simulink model "MidEval3"  (R2022b)
settings: Solver=VariableStepAuto  StartTime=0.0  StopTime=10.0  MaxStep=1e-3  RelTol=1e-4
model workspace (MAT data in the model file):
  DataStore = Simulink.Parameter
  DataStore.Value = [1 0 0 1 0 0 0 1 1 0 0 1 ... (2240 elements, 2240x1)]
  DataStore.DataType = 'auto'
  DataStore.Complexity = 'real'
  DataStore.Dimensions = [2240 1]
  Freq = Simulink.Parameter
  Freq.Value = 2000
  Freq.DataType = 'auto'
  Freq.Complexity = 'real'
  Freq.Dimensions = [1 1]
  Freq2 = Simulink.Parameter
  Freq2.Value = 6000000
  Freq2.DataType = 'auto'
  Freq2.Complexity = 'real'
  Freq2.Dimensions = [1 1]
  Freq3 = Simulink.Parameter
  Freq3.Value = 3000000
  Freq3.DataType = 'auto'
  Freq3.Complexity = 'real'
  Freq3.Dimensions = [1 1]
  Freq4 = Simulink.Parameter
  Freq4.Value = 10000000
  Freq4.DataType = 'auto'
  Freq4.Complexity = 'real'
  Freq4.Dimensions = [1 1]
  PreambleBits = Simulink.Parameter
  PreambleBits.Value = [1 1 1 1 1 0 0 1 1 0 1 0 1 1 1 1 1 1 0 0 1 1 0 1 0 1]
  PreambleBits.DataType = 'auto'
  PreambleBits.Complexity = 'real'
  PreambleBits.Dimensions = [1 26]
  fsr = 20
libraries: hdlsllib x4, simulink x2, commdigbbndam3 x2, dspfdesign x2
settings Model: Creator=Ceribro  LastModifiedBy=Ceribro

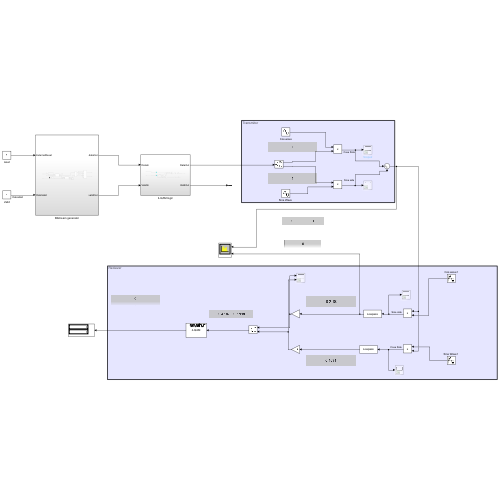
[thumbnail: Simulink's stored preview of the top-level diagram]
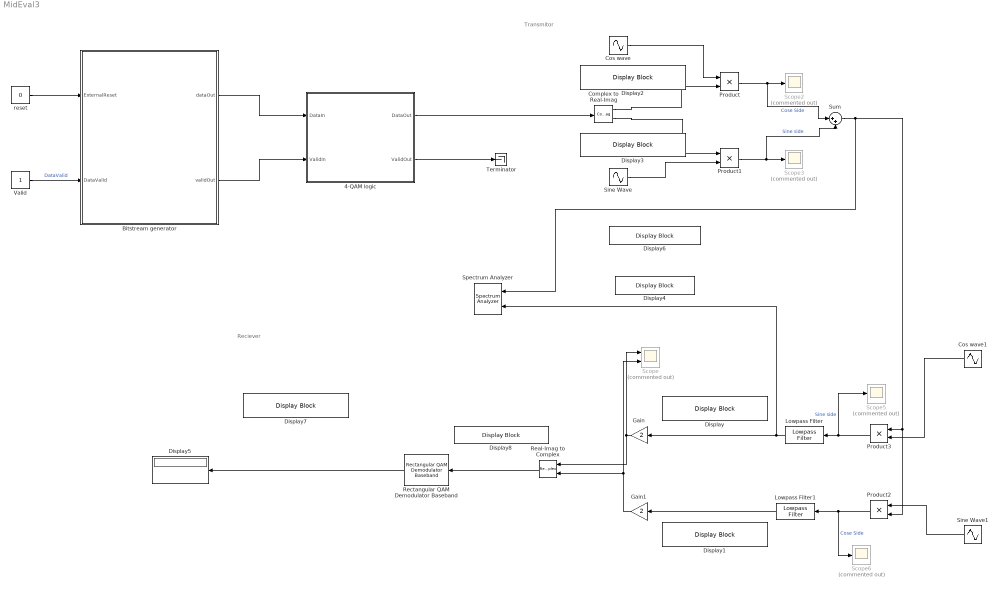
== system MidEval3 ==
  note: Reciever
  note: Transmitor
  4-QAM logic : Subsystem
  Bitstream generator : Subsystem
  Complex to Real-Imag : ComplexToRealImag
  Cos wave : Sin  Frequency=2*pi*Freq  Phase=pi/2  SampleTime=1/44100  VectorParams1D=off
  Cos wave1 : Sin  Frequency=2*pi*Freq  Phase=pi/2  SampleTime=1/44100  VectorParams1D=off
  Display{,1..4,6..8} (8 alike) : DisplayBlock  LabelPosition=Hide  Transparency=1
  Display5 : Display
  Gain : Gain  Gain=2
  Gain1 : Gain  Gain=2
  Lowpass Filter : dspfdesign/Lowpass Filter  FilterType=FIR  DesignForMinimumOrder=on  FilterOrder=50  PassbandFrequency=0.5e3  StopbandFrequency=1e3  PassbandRipple=0.1  StopbandAttenuation=80  InheritSampleRate=off  SampleRate=44100  SimulateUsing=Interpreted execution  roundingMode=Floor  coeffsDataTypeStr=fixdt(1,16)
  Lowpass Filter1 : dspfdesign/Lowpass Filter  FilterType=FIR  DesignForMinimumOrder=on  FilterOrder=50  PassbandFrequency=0.5e3  StopbandFrequency=1e3  PassbandRipple=0.1  StopbandAttenuation=80  InheritSampleRate=off  SampleRate=44100  SimulateUsing=Interpreted execution  roundingMode=Floor  coeffsDataTypeStr=fixdt(1,16)
  Product{,1..3} (4 alike) : Product
  Real-Imag to Complex : RealImagToComplex
  Rectangular QAM Demodulator Baseband : commdigbbndam3/Rectangular QAM Demodulator Baseband  M=4  OutType=Bit  DecType=Hard decision  VarSource=Dialog  Variance=1  Dec=Binary  Mapping=[0:15]  PowType=Min. distance between symbols  MinDist=2  AvgPow=1  PeakPow=1  Ph=0  outDtype1=Inherit via internal rule  outDtype2=Inherit via internal rule  derotateFactorWordLen=16  derotateFactorDataTypeStr=Inherit: Same word length as input  derotateFactorLastDataTypeStr=Inherit: Same word length as input  denormFactorWordLen=16  denormFactorDataTypeStr=Inherit: Same word length as input  denormFactorLastDataTypeStr=Inherit: Same word length as input  prodOutWordLen=32  prodOutOverflowMode=Wrap  prodOutRoundingMode=Floor  prodOutOvFlMode=off  prodOutOvFlModeLastStrValue=off  sumWordLen=32
      settings: LibrarySourceBlock=|
      | commhdldigbbndam/Rectangular QAM
      | Demodulator
      | Baseband
  Scope : Scope  Commented=on  NumInputPorts=2
  Scope{2..3,5..6} (4 alike) : Scope  Commented=on
  "Sine Wave " : Sin  Frequency=2*pi*Freq  SampleTime=1/44100  VectorParams1D=off
  "Sine Wave1 " : Sin  Frequency=2*pi*Freq  SampleTime=1/44100
  Spectrum Analyzer : SpectrumAnalyzer  NumInputPorts=2
  Sum : Sum  Inputs=|++
  Terminator : Terminator
  Valid : Constant  OutDataTypeStr=boolean  SampleTime=1/44100
  reset : Constant  Value=0  OutDataTypeStr=boolean
  wires:
  Rectangular QAM Demodulator Baseband/1 -> Display5/1
  Complex to Real-Imag/2 -> Product1/1
  Cos wave/1 -> Product/1
  "Sine Wave "/1 -> Product1/2
  Complex to Real-Imag/1 -> Product/2
  Product1/1 -> Scope3/1, Sum/2  "Sine side"
  Product/1 -> Scope2/1, Sum/1  "Cose Side"
  Lowpass Filter1/1 -> Gain1/1
  Product2/1 -> Lowpass Filter1/1, Scope6/1  "Cose Side"
  Lowpass Filter/1 -> Spectrum Analyzer/2, Gain/1
  Sum/1 -> Product2/2, Product3/1, Spectrum Analyzer/1
  Product3/1 -> Lowpass Filter/1, Scope5/1  "Sine side"
  Real-Imag to Complex/1 -> Rectangular QAM Demodulator Baseband/1
  Gain1/1 -> Real-Imag to Complex/2, Scope/2
  Gain/1 -> Scope/1, Real-Imag to Complex/1
  "Sine Wave1 "/1 -> Product2/1
  Cos wave1/1 -> Product3/2
  reset/1 -> Bitstream generator/1(ExternalReset)
  Valid/1 -> Bitstream generator/2(DataValid)  "DataValid"
  Bitstream generator/1(dataOut) -> 4-QAM logic/1(DataIn)
  Bitstream generator/2(validOut) -> 4-QAM logic/2(ValidIn)
  4-QAM logic/1(DataOut) -> Complex to Real-Imag/1
  4-QAM logic/2(ValidOut) -> Terminator/1

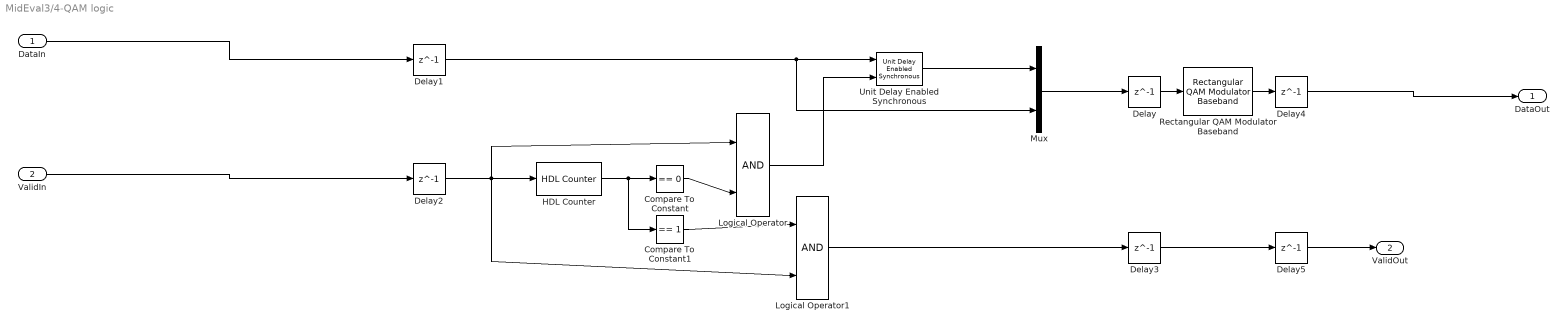
== system MidEval3/4-QAM logic ==
  DataIn : Inport
  ValidIn : Inport  Port=2
  Compare To Constant : simulink/Logic and Bit Operations/Compare To Constant  relop===  const=0  OutDataTypeStr=boolean
  Compare To Constant1 : simulink/Logic and Bit Operations/Compare To Constant  relop===  const=1  OutDataTypeStr=boolean
  Delay{,3..5} (4 alike) : Delay  DelayLength=1  InitialCondition=0
  Delay1 : Delay  DelayLength=1
  Delay2 : Delay  DelayLength=1
  HDL Counter : hdlsllib/Sources/HDL Counter  CountType=Count limited  CountInit=0  CountStep=1  CountMax=1  CountFromType=Initial value  CountFrom=0  CountResetPort=off  CountLoadPort=off  CountEnbPort=on  CountDirPort=off  CountHitOutputPort=off  CountDataType=Unsigned  CountWordLen=1  CountFracLen=0  CountSampTime=1
  Logical Operator : Logic  IconShape=distinctive  AllPortsSameDT=off  OutDataTypeStr=boolean
  Logical Operator1 : Logic  IconShape=distinctive  AllPortsSameDT=off  OutDataTypeStr=boolean
  Mux : Mux  Inputs=2
  Rectangular QAM Modulator Baseband : commdigbbndam3/Rectangular QAM Modulator Baseband  M=4  InType=Bit  Enc=Binary  Mapping=[0:15]  PowType=Min. distance between symbols  MinDist=2  AvgPow=1  PeakPow=1  Ph=0  outDtype=Fixed-point  outWordLen=16  outUDDataType=sfix(16)  outFracLenMode=User-defined  outFracLen=0  outDataTypeStr=fixdt(1,16,0)  outLastDataTypeStr=fixdt(1,16,0)
      settings: LibrarySourceBlock=|
      | commhdldigbbndam/Rectangular QAM
      | Modulator
      | Baseband
  Unit Delay Enabled Synchronous : hdlsllib/Discrete/Unit Delay Enabled Synchronous  InitialCondition=0.0  SampleTime=-1
  DataOut : Outport
  ValidOut : Outport  Port=2
  wires:
  Mux/1 -> Delay/1
  Delay1/1 -> Mux/2, Unit Delay Enabled Synchronous/1
  Logical Operator/1 -> Unit Delay Enabled Synchronous/2
  Delay5/1 -> ValidOut/1
  Delay2/1 -> HDL Counter/1, Logical Operator/1, Logical Operator1/2
  Compare To Constant/1 -> Logical Operator/2
  Rectangular QAM Modulator Baseband/1 -> Delay4/1
  Unit Delay Enabled Synchronous/1 -> Mux/1
  Compare To Constant1/1 -> Logical Operator1/1
  HDL Counter/1 -> Compare To Constant1/1, Compare To Constant/1
  Logical Operator1/1 -> Delay3/1
  Delay3/1 -> Delay5/1
  Delay/1 -> Rectangular QAM Modulator Baseband/1
  Delay4/1 -> DataOut/1
  ValidIn/1 -> Delay2/1
  DataIn/1 -> Delay1/1

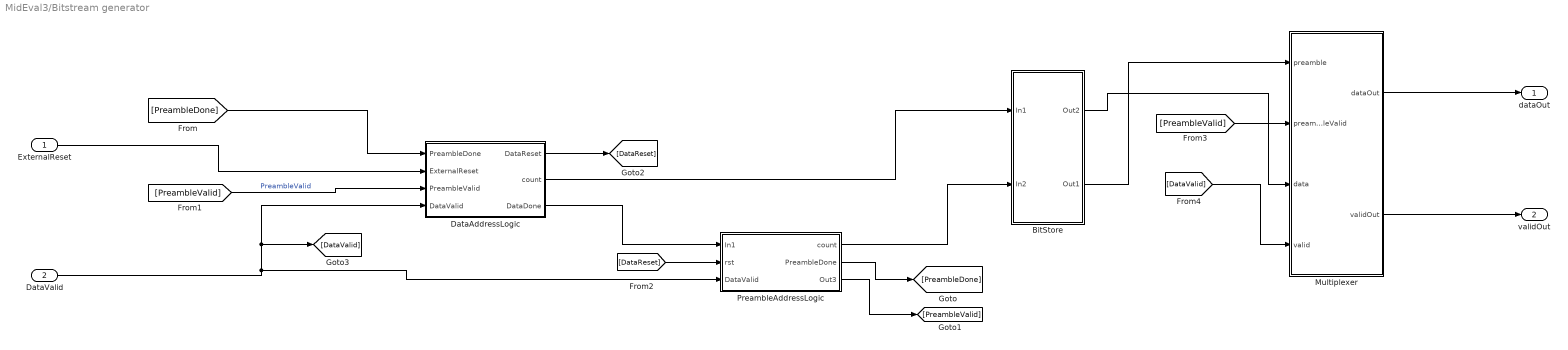
== system MidEval3/Bitstream generator ==
  ExternalReset : Inport
  DataValid : Inport  Port=2
  BitStore : Subsystem
  DataAddressLogic : Subsystem
  Multiplexer : Subsystem
  PreambleAddressLogic : Subsystem
  dataOut : Outport
  validOut : Outport  Port=2
  wires:
  BitStore/2(Out1) -> Multiplexer/1(preamble)
  DataValid/1 -> [DataValid], DataAddressLogic/4(DataValid), PreambleAddressLogic/3(DataValid)
  DataAddressLogic/2(count) -> BitStore/1(In1)
  DataAddressLogic/3(DataDone) -> PreambleAddressLogic/1(In1)
  [DataReset] -> PreambleAddressLogic/2(rst)
  PreambleAddressLogic/1(count) -> BitStore/2(In2)
  [DataValid] -> Multiplexer/4(valid)
  PreambleAddressLogic/2(PreambleDone) -> [PreambleDone]
  [PreambleDone] -> DataAddressLogic/1(PreambleDone)
  PreambleAddressLogic/3(Out3) -> [PreambleValid]
  [PreambleValid] -> Multiplexer/2(preambleValid)
  BitStore/1(Out2) -> Multiplexer/3(data)
  DataAddressLogic/1(DataReset) -> [DataReset]
  ExternalReset/1 -> DataAddressLogic/2(ExternalReset)
  [PreambleValid] -> DataAddressLogic/3(PreambleValid)  "PreambleValid"
  Multiplexer/1(dataOut) -> dataOut/1
  Multiplexer/2(validOut) -> validOut/1

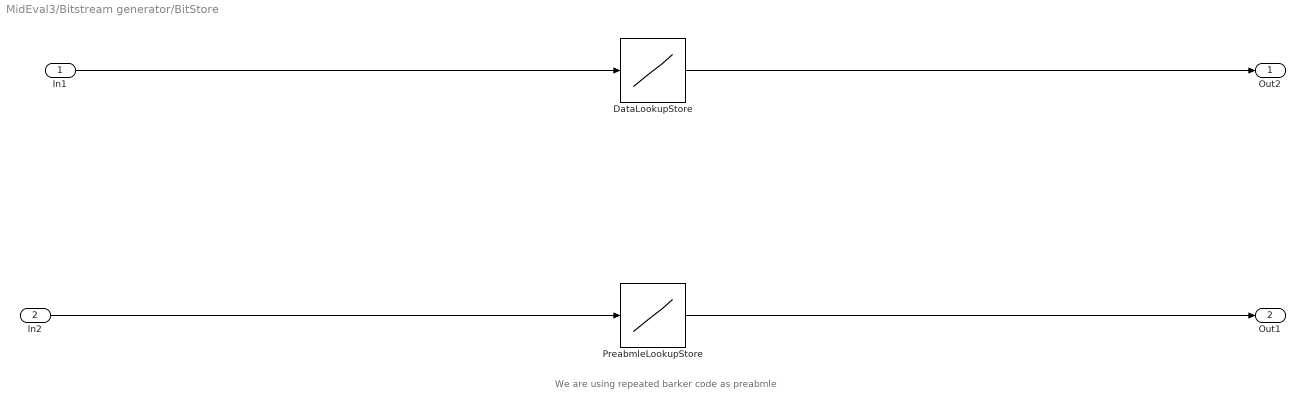
== system MidEval3/Bitstream generator/BitStore ==
  note: We are using repeated barker code as preabmle
  In1 : Inport
  In2 : Inport  Port=2
  DataLookupStore : Lookup_n-D  NumberOfTableDimensions=1  LookupTableObject=''  BreakpointsForDimension1=0:length(DataStore)-1  BreakpointsForDimension1FirstPoint=10  BreakpointsForDimension2FirstPoint=10  BreakpointsForDimension1Spacing=12  BreakpointsForDimension2Spacing=12  IndexSearchMethod=Evenly spaced points  Table=DataStore  TableDataTypeStr=single  InterpMethod=Flat  DiagnosticForOutOfRangeInput=Error  InternalRulePriority=Speed  OutDataTypeStr=single  RndMeth=Simplest
  PreabmleLookupStore : Lookup_n-D  NumberOfTableDimensions=1  BreakpointsForDimension1=0:length(PreambleBits)-1  IndexSearchMethod=Evenly spaced points  Table=PreambleBits  TableDataTypeStr=single  InterpMethod=Flat  DiagnosticForOutOfRangeInput=Error  InternalRulePriority=Speed  OutDataTypeStr=single  RndMeth=Simplest
  Out2 : Outport
  Out1 : Outport  Port=2
  wires:
  In2/1 -> PreabmleLookupStore/1
  DataLookupStore/1 -> Out2/1
  PreabmleLookupStore/1 -> Out1/1
  In1/1 -> DataLookupStore/1

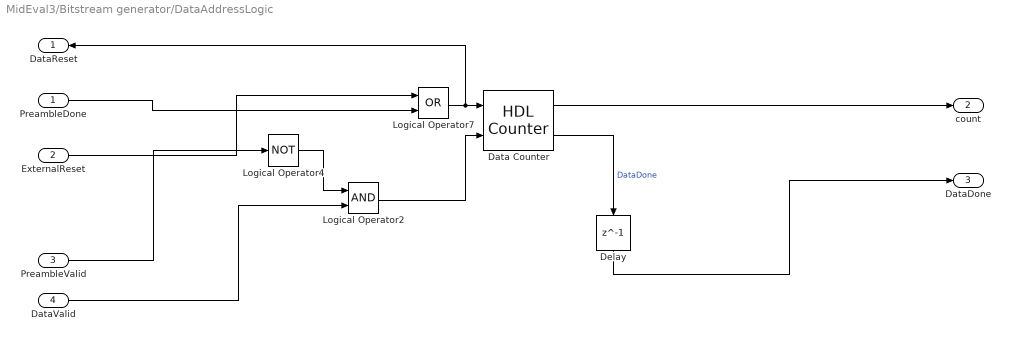
== system MidEval3/Bitstream generator/DataAddressLogic ==
  PreambleDone : Inport
  ExternalReset : Inport  Port=2
  PreambleValid : Inport  Port=3
  DataValid : Inport  Port=4
  Data Counter : hdlsllib/Sources/HDL Counter  CountType=Count limited  CountInit=0  CountStep=1  CountMax=length(DataStore)-1  CountFromType=Specify  CountFrom=0  CountResetPort=on  CountLoadPort=off  CountEnbPort=on  CountDirPort=off  CountHitOutputPort=on  CountDataType=Unsigned  CountWordLen=nextpow2(length(DataStore)-1)  CountFracLen=0  CountSampTime=1
  Delay : Delay  DelayLength=1  InitialCondition=0
  Logical Operator2 : Logic  AllPortsSameDT=off  OutDataTypeStr=boolean
  Logical Operator4 : Logic  Operator=NOT  AllPortsSameDT=off  OutDataTypeStr=boolean
  Logical Operator7 : Logic  Operator=OR  AllPortsSameDT=off  OutDataTypeStr=boolean
  DataReset : Outport
  count : Outport  Port=2
  DataDone : Outport  Port=3
  wires:
  PreambleDone/1 -> Logical Operator7/2
  DataValid/1 -> Logical Operator2/2
  Logical Operator2/1 -> Data Counter/2
  Logical Operator4/1 -> Logical Operator2/1
  ExternalReset/1 -> Logical Operator7/1
  Data Counter/2 -> Delay/1  "DataDone"
  Logical Operator7/1 -> DataReset/1, Data Counter/1
  PreambleValid/1 -> Logical Operator4/1
  Data Counter/1 -> count/1
  Delay/1 -> DataDone/1

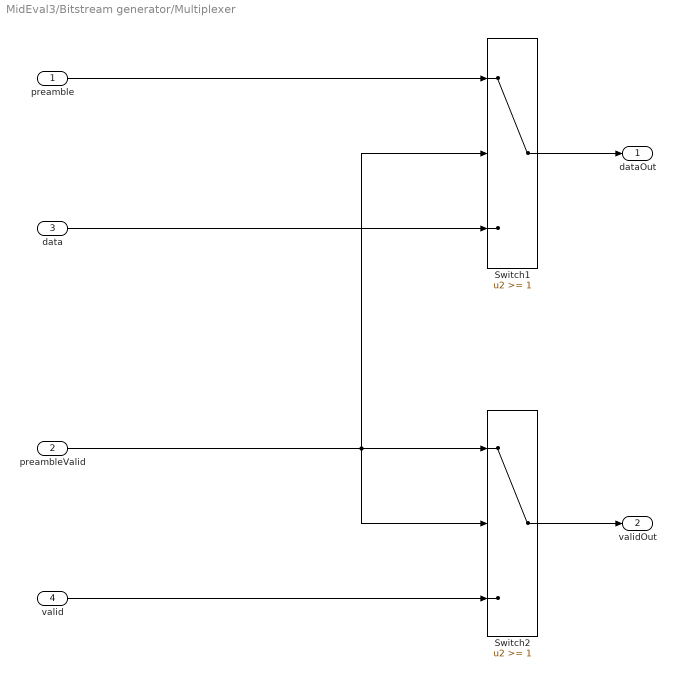
== system MidEval3/Bitstream generator/Multiplexer ==
  preamble : Inport
  preambleValid : Inport  Port=2
  data : Inport  Port=3
  valid : Inport  Port=4
  Switch1 : Switch  Threshold=1  SaturateOnIntegerOverflow=off  InputSameDT=off
  Switch2 : Switch  Threshold=1  SaturateOnIntegerOverflow=off  InputSameDT=off
  dataOut : Outport
  validOut : Outport  Port=2
  wires:
  Switch2/1 -> validOut/1
  Switch1/1 -> dataOut/1
  valid/1 -> Switch2/3
  preambleValid/1 -> Switch1/2, Switch2/2, Switch2/1
  preamble/1 -> Switch1/1
  data/1 -> Switch1/3

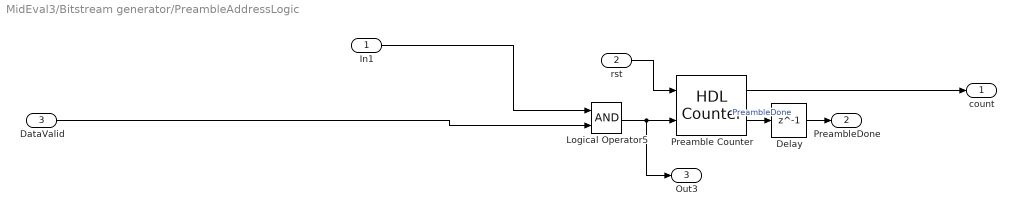
== system MidEval3/Bitstream generator/PreambleAddressLogic ==
  In1 : Inport
  rst : Inport  Port=2
  DataValid : Inport  Port=3
  Delay : Delay  DelayLength=1  InitialCondition=0
  Logical Operator5 : Logic  AllPortsSameDT=off  OutDataTypeStr=boolean
  Preamble Counter : hdlsllib/Sources/HDL Counter  CountType=Count limited  CountInit=0  CountStep=1  CountMax=length(DataStore)-1  CountFromType=Specify  CountFrom=0  CountResetPort=on  CountLoadPort=off  CountEnbPort=on  CountDirPort=off  CountHitOutputPort=on  CountDataType=Unsigned  CountWordLen=nextpow2(length(DataStore)-1)  CountFracLen=0  CountSampTime=1
  count : Outport
  PreambleDone : Outport  Port=2
  Out3 : Outport  Port=3
  wires:
  Logical Operator5/1 -> Out3/1, Preamble Counter/2
  Preamble Counter/1 -> count/1
  DataValid/1 -> Logical Operator5/2
  In1/1 -> Logical Operator5/1
  Preamble Counter/2 -> Delay/1  "PreambleDone"
  rst/1 -> Preamble Counter/1
  Delay/1 -> PreambleDone/1
